simulink model "simularePIdiscret"  (R2022b)
settings: Solver=VariableStepAuto  StartTime=0.0  StopTime=25  RelTol=1e-3
values from neighbouring files (symbols this model uses):
  A = Hd.den{1}    [VariantaBUNA10.m]
  Ar = Hrdiscret.den{1}    [VariantaBUNA10.m]
  B = Hd.num{1}    [VariantaBUNA10.m]
  Br = Hrdiscret.num{1}    [VariantaBUNA10.m]
settings Model: Creator=saioc  LastModifiedBy=saioc
settings ModelReferenceCC: EnableRefExpFcnMdlSchedulingChecks=on

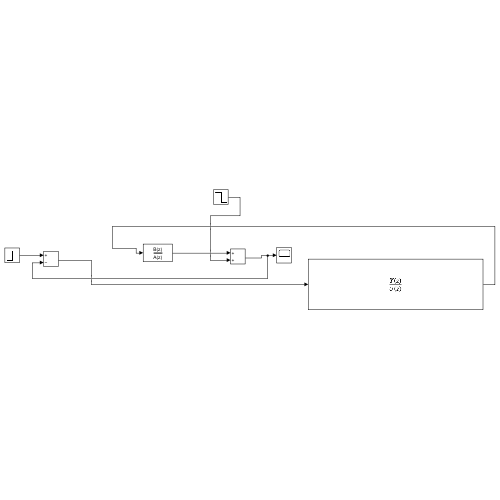
[thumbnail: Simulink's stored preview of the top-level diagram]
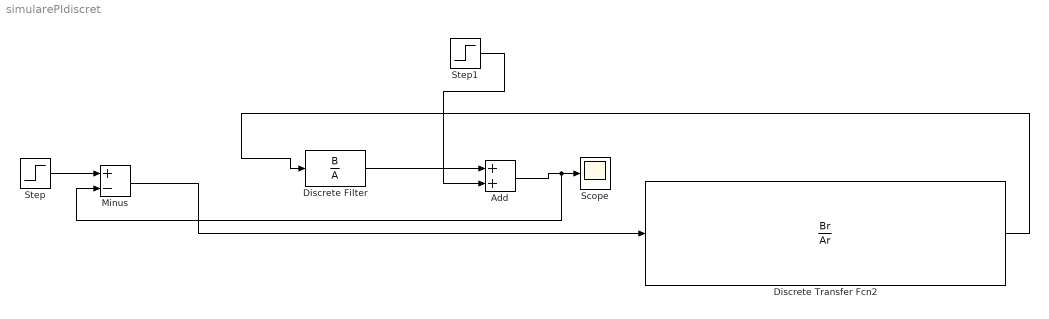
== system simularePIdiscret ==
  Add : Sum
  Discrete Transfer Fcn2 : DiscreteTransferFcn  Numerator=Br  Denominator=Ar  SampleTime=0.1
  Discrete Filter : DiscreteFilter  Numerator=B  Denominator=A  SampleTime=0.1
  Minus : Sum  Inputs=+-
  Scope : Scope
  Step : Step  After=150  SampleTime=0.1
  Step1 : Step  Time=9  After=-100  SampleTime=0.1
  wires:
  Discrete Filter/1 -> Add/1
  Add/1 -> Minus/2, Scope/1
  Step/1 -> Minus/1
  Minus/1 -> Discrete Transfer Fcn2/1
  Discrete Transfer Fcn2/1 -> Discrete Filter/1
  Step1/1 -> Add/2
